simulink model "Punto3"  (R2024b)
settings: Solver=VariableStepAuto  StartTime=0.0  StopTime=20  RelTol=1e-3
libraries: simulink x2
settings Model: Creator=Andres Felipe  LastModifiedBy=Andres Felipe

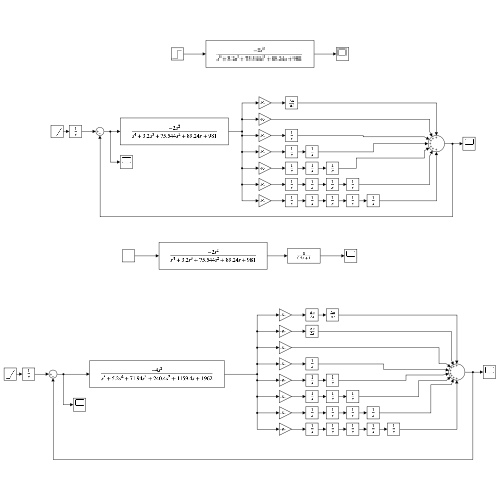
[thumbnail: Simulink's stored preview of the top-level diagram]
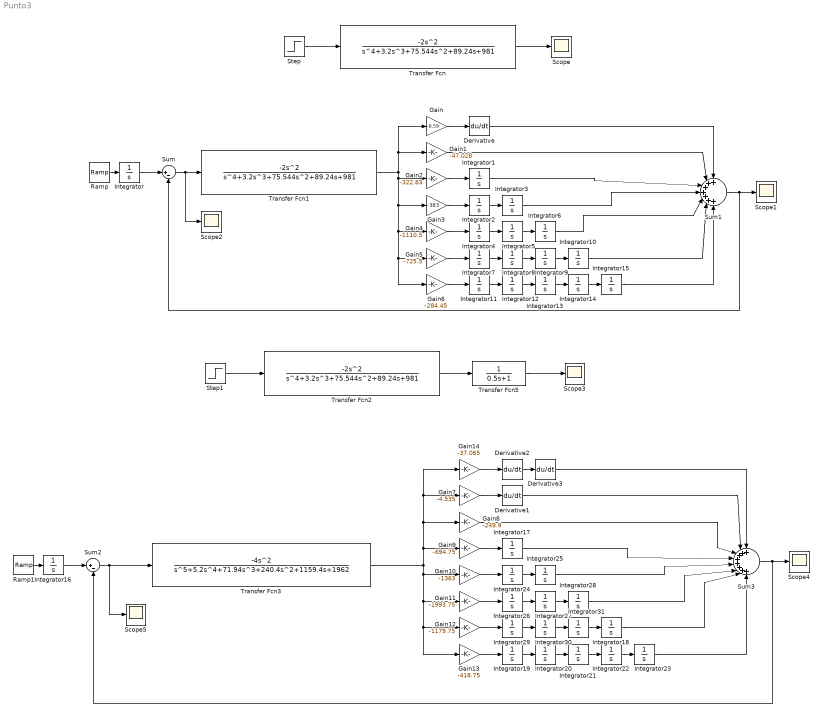
== system Punto3 ==
  Derivative{,1..3} (4 alike) : Derivative
  Gain : Gain  Gain=-8.59
  Gain1 : Gain  Gain=-47.028
  Gain10 : Gain  Gain=-1363
  Gain11 : Gain  Gain=-1993.75
  Gain12 : Gain  Gain=-1179.75
  Gain13 : Gain  Gain=-418.75
  Gain14 : Gain  Gain=-37.065
  Gain2 : Gain  Gain=-322.83
  Gain3 : Gain  Gain=-383
  Gain4 : Gain  Gain=-1110.5
  Gain5 : Gain  Gain=-725.5
  Gain6 : Gain  Gain=-284.45
  Gain7 : Gain  Gain=-4.535
  Gain8 : Gain  Gain=-249.9
  Gain9 : Gain  Gain=-694.75
  Integrator{,1..31} (32 alike) : Integrator
  Ramp : simulink/Sources/Ramp  slope=1  start=0  InitialOutput=0
  Ramp1 : simulink/Sources/Ramp  slope=1  start=0  InitialOutput=0
  Scope{,1..5} (6 alike) : Scope
  Step : Step  Time=0  SampleTime=0
  Step1 : Step  Time=0  SampleTime=0
  Sum : Sum  Inputs=|+-
  Sum1 : Sum  Inputs=+++++++
  Sum2 : Sum  Inputs=|+-
  Sum3 : Sum  Inputs=++++++++
  Transfer Fcn : TransferFcn  Numerator=[-2 0 0]  Denominator=[1 3.2 75.544 89.24 981]
  Transfer Fcn1 : TransferFcn  Numerator=[-2 0 0]  Denominator=[1 3.2 75.544 89.24 981]
  Transfer Fcn2 : TransferFcn  Numerator=[-2 0 0]  Denominator=[1 3.2 75.544 89.24 981]
  Transfer Fcn3 : TransferFcn  Numerator=[-4 0 0]  Denominator=[1 5.2 71.94 240.4 1159.4 1962]
  Transfer Fcn5 : TransferFcn  Denominator=[0.5 1]
  wires:
  Step/1 -> Transfer Fcn/1
  Transfer Fcn/1 -> Scope/1
  Ramp/1 -> Integrator/1
  Integrator/1 -> Sum/1
  Sum/1 -> Scope2/1, Transfer Fcn1/1
  Sum1/1 -> Sum/2, Scope1/1
  Integrator2/1 -> Integrator3/1
  Integrator4/1 -> Integrator5/1
  Integrator5/1 -> Integrator6/1
  Integrator8/1 -> Integrator9/1
  Integrator9/1 -> Integrator10/1
  Integrator7/1 -> Integrator8/1
  Integrator13/1 -> Integrator14/1
  Integrator14/1 -> Integrator15/1
  Integrator11/1 -> Integrator12/1
  Integrator12/1 -> Integrator13/1
  Gain6/1 -> Integrator11/1
  Gain5/1 -> Integrator7/1
  Gain4/1 -> Integrator4/1
  Gain3/1 -> Integrator2/1
  Gain2/1 -> Integrator1/1
  Gain/1 -> Derivative/1
  Transfer Fcn1/1 -> Gain6/1, Gain5/1, Gain4/1, Gain3/1, Gain2/1, Gain/1, Gain1/1
  Derivative/1 -> Sum1/1
  Gain1/1 -> Sum1/2
  Integrator1/1 -> Sum1/3
  Integrator3/1 -> Sum1/4
  Integrator6/1 -> Sum1/5
  Integrator10/1 -> Sum1/6
  Integrator15/1 -> Sum1/7
  Transfer Fcn5/1 -> Scope3/1
  Step1/1 -> Transfer Fcn2/1
  Integrator23/1 -> Sum3/8
  Sum3/1 -> Sum2/2, Scope4/1
  Integrator28/1 -> Sum3/6
  Gain7/1 -> Derivative1/1
  Derivative1/1 -> Sum3/2
  Gain8/1 -> Sum3/3
  Integrator18/1 -> Sum3/7
  Gain13/1 -> Integrator19/1
  Integrator31/1 -> Integrator18/1
  Sum2/1 -> Transfer Fcn3/1, Scope5/1
  Ramp1/1 -> Integrator16/1
  Integrator26/1 -> Integrator27/1
  Integrator17/1 -> Sum3/4
  Integrator16/1 -> Sum2/1
  Gain10/1 -> Integrator24/1
  Integrator20/1 -> Integrator21/1
  Gain9/1 -> Integrator17/1
  Integrator30/1 -> Integrator31/1
  Integrator21/1 -> Integrator22/1
  Integrator25/1 -> Sum3/5
  Gain12/1 -> Integrator29/1
  Integrator19/1 -> Integrator20/1
  Integrator24/1 -> Integrator25/1
  Integrator27/1 -> Integrator28/1
  Integrator22/1 -> Integrator23/1
  Integrator29/1 -> Integrator30/1
  Gain11/1 -> Integrator26/1
  Transfer Fcn3/1 -> Gain13/1, Gain12/1, Gain11/1, Gain10/1, Gain14/1, Gain7/1, Gain8/1, Gain9/1
  Transfer Fcn2/1 -> Transfer Fcn5/1
  Derivative2/1 -> Derivative3/1
  Gain14/1 -> Derivative2/1
  Derivative3/1 -> Sum3/1
